simulink model "ALL_JP360_DBW_V6_5_1103"  (R2022a)
settings: Solver=FixedStepAuto  StartTime=0.0  StopTime=inf  FixedStep=0.01  RelTol=1e-3  EnableMultiTasking=on
model workspace (MAT data in the model file):
  g = 9.8
undefined symbols (not defined in the file or in its folder): canChannel, delta_v_p, IPM_Line_C0, IPM_Line_C1, IPM_Line_C2, IPM_Line_C3, M, M_p, MRR_ObjDistX, MRR_ObjDistY, MRR_ObjFusionCamID, MRR_ObjFusionSig, MRR_ObjID, MRR_ObjRelVelX, MRR_ObjRelVelY, MRR_ObjType, MRR_ObjUpdFlg, none, obj_vaild, untracktime, V, videoinput
libraries: canfdmsglib x230, canfdlib x76, slpidlib x24, simulink x18, dspstat3 x14, ctrlSharedLib x1, simulink_extras x1, imaqlib x1, realtime_pacer_lib x1, dspvision x1, visionsinks x1
(part 44 of 55)

== system ALL_JP360_DBW_V6_5_1103/MsgFromCAN/VR_ADCU_MsgFromCAN/VR_ADCU_IPM_Obj_13_0x65C ==
  VR_ADCU_IPM_Obj_13_0x65CFromInData : Inport  OutDataTypeStr=Bus:CAN_FD_MESSAGE_BUS
  Bus Creator : BusCreator  Inputs=18  OutDataTypeStr=Bus:VR_ADCU_IPM_Obj_13_0x65C  NonVirtualBus=on
  CAN FD Unpack : canfdmsglib/CAN FD Unpack  CANdbFile=HiFire_T360_P789_1R1V_Pri_Matrix_CAN_V2.3_20220810.dbc  MsgList=(none)  MsgName=IPM_Obj_13_0x65C  ProtocolMode=CAN FD  MsgIDType=Standard (11-bit identifier)  MsgIdentifier=1628  MsgLength=32  SignalInfo={'IPM_ObjBlockCounter_13','13','11','BE','unsigned','Standard','0','1','0','0','2047';'IPM_ObjDistX_13','58','12','BE','unsigned','Standard','0','0.0625','0','0','254.9375';'IPM_ObjDistY_13','76','14','BE','unsigned','Standard','0','0.0078125','-64','-64','63.9922';'IPM_ObjID_13','16','8','BE','unsigned','Standard','0','1','0','0','255';'IPM_ObjRelAccelX_13','104','10','BE','unsigned','Standard','0','0.03125','-16','-16','15.9688';'IPM_ObjRelAccelY_13','126','10','BE','unsigned','Standard','0','0.03125','-16','-16','15.9688';'IPM_ObjRelVelX_13','95','13','BE','unsigned','Standard','0','0.03125','-128','-128','127.9688';'IPM_ObjRelVelY_13','98','13','BE','unsigned','Standard','0','0.03125','-128','-128','127.9688';'IPM_ObjType_13','54','4','BE','unsigned','Standard','0','1','0','0','15';'IPM_Obj_13_Checksum','248','16','BE','unsigned','Standard','0','1','0','0','65535';'IPM_Obj_13_MsgCounter','232','4','BE','unsigned','Standard','0','1','0','0','15';'IPM_Object_Age_13','37','11','BE','unsigned','Standard','0','1','0','0','2047';'IPM_Object_Existence_Probability_13','42','6','BE','unsigned','Standard','0','2','0','0','100';'IPM_Object_Heading_13','132','10','BE','unsigned','Standard','0','0.01','-3.14','-3.14','3.14';'IPM_Object_Height_13','167','9','BE','unsigned','Standard','0','0.01','0','0','5.11';'IPM_Object_Length_13','139','9','BE','unsigned','Standard','0','0.05','0','0','25.5';'IPM_Object_Motion_Status_13','161','3','BE','unsigned','Standard','0','1','0','0','7';'IPM_Object_Width_13','144','11','BE','unsigned','Standard','0','0.01','0','0','12'}  IDPort=off  TimestampPort=off  ErrorPort=off  RemotePort=off  LengthPort=off  StatusPort=off  BRSPort=off  ESIPort=off  DLCPort=off  ApplyMinMax=off
      settings: SourceProductBaseCode=ME,XP,VN  DataFormat=CANdb specified signals
  Data Type Conversion1 : DataTypeConversion  OutDataTypeStr=int16  SaturateOnIntegerOverflow=off  RndMeth=Floor
  Data Type Conversion10 : DataTypeConversion  OutDataTypeStr=uint16  SaturateOnIntegerOverflow=off  RndMeth=Floor
  Data Type Conversion{9,11,13,17} (4 alike) : DataTypeConversion  OutDataTypeStr=int8  SaturateOnIntegerOverflow=off  RndMeth=Floor
  Data Type Conversion12 : DataTypeConversion  OutDataTypeStr=int16  SaturateOnIntegerOverflow=off  RndMeth=Floor
  Data Type Conversion{2..3,5..8,14..16,18} (10 alike) : DataTypeConversion  OutDataTypeStr=single  SaturateOnIntegerOverflow=off  RndMeth=Floor
  Data Type Conversion4 : DataTypeConversion  OutDataTypeStr=uint8  SaturateOnIntegerOverflow=off  RndMeth=Floor
  VR_ADCU_IPM_Obj_13_0x65CFromOutData : Outport  OutDataTypeStr=Bus:VR_ADCU_IPM_Obj_13_0x65C
  wires:
  CAN FD Unpack/1 -> Data Type Conversion1/1
  CAN FD Unpack/2 -> Data Type Conversion2/1
  CAN FD Unpack/3 -> Data Type Conversion3/1
  CAN FD Unpack/4 -> Data Type Conversion4/1
  CAN FD Unpack/5 -> Data Type Conversion5/1
  CAN FD Unpack/6 -> Data Type Conversion6/1
  CAN FD Unpack/7 -> Data Type Conversion7/1
  CAN FD Unpack/8 -> Data Type Conversion8/1
  CAN FD Unpack/9 -> Data Type Conversion9/1
  CAN FD Unpack/10 -> Data Type Conversion10/1
  CAN FD Unpack/11 -> Data Type Conversion11/1
  CAN FD Unpack/12 -> Data Type Conversion12/1
  CAN FD Unpack/13 -> Data Type Conversion13/1
  CAN FD Unpack/14 -> Data Type Conversion14/1
  CAN FD Unpack/15 -> Data Type Conversion15/1
  CAN FD Unpack/16 -> Data Type Conversion16/1
  CAN FD Unpack/17 -> Data Type Conversion17/1
  CAN FD Unpack/18 -> Data Type Conversion18/1
  Data Type Conversion1/1 -> Bus Creator/1  "IPM_ObjBlockCounter_13"
  Data Type Conversion2/1 -> Bus Creator/2  "IPM_ObjDistX_13"
  Data Type Conversion3/1 -> Bus Creator/3  "IPM_ObjDistY_13"
  Data Type Conversion4/1 -> Bus Creator/4  "IPM_ObjID_13"
  Data Type Conversion5/1 -> Bus Creator/5  "IPM_ObjRelAccelX_13"
  Data Type Conversion6/1 -> Bus Creator/6  "IPM_ObjRelAccelY_13"
  Data Type Conversion7/1 -> Bus Creator/7  "IPM_ObjRelVelX_13"
  Data Type Conversion8/1 -> Bus Creator/8  "IPM_ObjRelVelY_13"
  Data Type Conversion9/1 -> Bus Creator/9  "IPM_ObjType_13"
  Data Type Conversion10/1 -> Bus Creator/10  "IPM_Obj_13_Checksum"
  Data Type Conversion11/1 -> Bus Creator/11  "IPM_Obj_13_MsgCounter"
  Data Type Conversion12/1 -> Bus Creator/12  "IPM_Object_Age_13"
  Data Type Conversion13/1 -> Bus Creator/13  "IPM_Object_Existence_Probability_13"
  Data Type Conversion14/1 -> Bus Creator/14  "IPM_Object_Heading_13"
  Data Type Conversion15/1 -> Bus Creator/15  "IPM_Object_Height_13"
  Data Type Conversion16/1 -> Bus Creator/16  "IPM_Object_Length_13"
  Data Type Conversion17/1 -> Bus Creator/17  "IPM_Object_Motion_Status_13"
  Data Type Conversion18/1 -> Bus Creator/18  "IPM_Object_Width_13"
  Bus Creator/1 -> VR_ADCU_IPM_Obj_13_0x65CFromOutData/1  "VR_ADCU_IPM_Obj_13_0x65CFromOutData"
  VR_ADCU_IPM_Obj_13_0x65CFromInData/1 -> CAN FD Unpack/1  "VR_ADCU_IPM_Obj_13_0x65CFromInData"

== system ALL_JP360_DBW_V6_5_1103/MsgFromCAN/VR_ADCU_MsgFromCAN/VR_ADCU_IPM_Obj_14_0x65D ==
  VR_ADCU_IPM_Obj_14_0x65DFromInData : Inport  OutDataTypeStr=Bus:CAN_FD_MESSAGE_BUS
  Bus Creator : BusCreator  Inputs=18  OutDataTypeStr=Bus:VR_ADCU_IPM_Obj_14_0x65D  NonVirtualBus=on
  CAN FD Unpack : canfdmsglib/CAN FD Unpack  CANdbFile=HiFire_T360_P789_1R1V_Pri_Matrix_CAN_V2.3_20220810.dbc  MsgList=(none)  MsgName=IPM_Obj_14_0x65D  ProtocolMode=CAN FD  MsgIDType=Standard (11-bit identifier)  MsgIdentifier=1629  MsgLength=32  SignalInfo={'IPM_ObjBlockCounter_14','13','11','BE','unsigned','Standard','0','1','0','0','2047';'IPM_ObjDistX_14','58','12','BE','unsigned','Standard','0','0.0625','0','0','254.9375';'IPM_ObjDistY_14','76','14','BE','unsigned','Standard','0','0.0078125','-64','-64','63.9922';'IPM_ObjID_14','16','8','BE','unsigned','Standard','0','1','0','0','255';'IPM_ObjRelAccelX_14','104','10','BE','unsigned','Standard','0','0.03125','-16','-16','15.9688';'IPM_ObjRelAccelY_14','126','10','BE','unsigned','Standard','0','0.03125','-16','-16','15.9688';'IPM_ObjRelVelX_14','95','13','BE','unsigned','Standard','0','0.03125','-128','-128','127.9688';'IPM_ObjRelVelY_14','98','13','BE','unsigned','Standard','0','0.03125','-128','-128','127.9688';'IPM_ObjType_14','54','4','BE','unsigned','Standard','0','1','0','0','15';'IPM_Obj_14_Checksum','248','16','BE','unsigned','Standard','0','1','0','0','65535';'IPM_Obj_14_MsgCounter','232','4','BE','unsigned','Standard','0','1','0','0','15';'IPM_Object_Age_14','37','11','BE','unsigned','Standard','0','1','0','0','2047';'IPM_Object_Existence_Probability_14','42','6','BE','unsigned','Standard','0','2','0','0','100';'IPM_Object_Heading_14','132','10','BE','unsigned','Standard','0','0.01','-3.14','-3.14','3.14';'IPM_Object_Height_14','167','9','BE','unsigned','Standard','0','0.01','0','0','5.11';'IPM_Object_Length_14','139','9','BE','unsigned','Standard','0','0.05','0','0','25.5';'IPM_Object_Motion_Status_14','161','3','BE','unsigned','Standard','0','1','0','0','7';'IPM_Object_Width_14','144','11','BE','unsigned','Standard','0','0.01','0','0','12'}  IDPort=off  TimestampPort=off  ErrorPort=off  RemotePort=off  LengthPort=off  StatusPort=off  BRSPort=off  ESIPort=off  DLCPort=off  ApplyMinMax=off
      settings: SourceProductBaseCode=ME,XP,VN  DataFormat=CANdb specified signals
  Data Type Conversion1 : DataTypeConversion  OutDataTypeStr=int16  SaturateOnIntegerOverflow=off  RndMeth=Floor
  Data Type Conversion10 : DataTypeConversion  OutDataTypeStr=uint16  SaturateOnIntegerOverflow=off  RndMeth=Floor
  Data Type Conversion{9,11,13,17} (4 alike) : DataTypeConversion  OutDataTypeStr=int8  SaturateOnIntegerOverflow=off  RndMeth=Floor
  Data Type Conversion12 : DataTypeConversion  OutDataTypeStr=int16  SaturateOnIntegerOverflow=off  RndMeth=Floor
  Data Type Conversion{2..3,5..8,14..16,18} (10 alike) : DataTypeConversion  OutDataTypeStr=single  SaturateOnIntegerOverflow=off  RndMeth=Floor
  Data Type Conversion4 : DataTypeConversion  OutDataTypeStr=uint8  SaturateOnIntegerOverflow=off  RndMeth=Floor
  VR_ADCU_IPM_Obj_14_0x65DFromOutData : Outport  OutDataTypeStr=Bus:VR_ADCU_IPM_Obj_14_0x65D
  wires:
  CAN FD Unpack/1 -> Data Type Conversion1/1
  CAN FD Unpack/2 -> Data Type Conversion2/1
  CAN FD Unpack/3 -> Data Type Conversion3/1
  CAN FD Unpack/4 -> Data Type Conversion4/1
  CAN FD Unpack/5 -> Data Type Conversion5/1
  CAN FD Unpack/6 -> Data Type Conversion6/1
  CAN FD Unpack/7 -> Data Type Conversion7/1
  CAN FD Unpack/8 -> Data Type Conversion8/1
  CAN FD Unpack/9 -> Data Type Conversion9/1
  CAN FD Unpack/10 -> Data Type Conversion10/1
  CAN FD Unpack/11 -> Data Type Conversion11/1
  CAN FD Unpack/12 -> Data Type Conversion12/1
  CAN FD Unpack/13 -> Data Type Conversion13/1
  CAN FD Unpack/14 -> Data Type Conversion14/1
  CAN FD Unpack/15 -> Data Type Conversion15/1
  CAN FD Unpack/16 -> Data Type Conversion16/1
  CAN FD Unpack/17 -> Data Type Conversion17/1
  CAN FD Unpack/18 -> Data Type Conversion18/1
  Data Type Conversion1/1 -> Bus Creator/1  "IPM_ObjBlockCounter_14"
  Data Type Conversion2/1 -> Bus Creator/2  "IPM_ObjDistX_14"
  Data Type Conversion3/1 -> Bus Creator/3  "IPM_ObjDistY_14"
  Data Type Conversion4/1 -> Bus Creator/4  "IPM_ObjID_14"
  Data Type Conversion5/1 -> Bus Creator/5  "IPM_ObjRelAccelX_14"
  Data Type Conversion6/1 -> Bus Creator/6  "IPM_ObjRelAccelY_14"
  Data Type Conversion7/1 -> Bus Creator/7  "IPM_ObjRelVelX_14"
  Data Type Conversion8/1 -> Bus Creator/8  "IPM_ObjRelVelY_14"
  Data Type Conversion9/1 -> Bus Creator/9  "IPM_ObjType_14"
  Data Type Conversion10/1 -> Bus Creator/10  "IPM_Obj_14_Checksum"
  Data Type Conversion11/1 -> Bus Creator/11  "IPM_Obj_14_MsgCounter"
  Data Type Conversion12/1 -> Bus Creator/12  "IPM_Object_Age_14"
  Data Type Conversion13/1 -> Bus Creator/13  "IPM_Object_Existence_Probability_14"
  Data Type Conversion14/1 -> Bus Creator/14  "IPM_Object_Heading_14"
  Data Type Conversion15/1 -> Bus Creator/15  "IPM_Object_Height_14"
  Data Type Conversion16/1 -> Bus Creator/16  "IPM_Object_Length_14"
  Data Type Conversion17/1 -> Bus Creator/17  "IPM_Object_Motion_Status_14"
  Data Type Conversion18/1 -> Bus Creator/18  "IPM_Object_Width_14"
  Bus Creator/1 -> VR_ADCU_IPM_Obj_14_0x65DFromOutData/1  "VR_ADCU_IPM_Obj_14_0x65DFromOutData"
  VR_ADCU_IPM_Obj_14_0x65DFromInData/1 -> CAN FD Unpack/1  "VR_ADCU_IPM_Obj_14_0x65DFromInData"

== system ALL_JP360_DBW_V6_5_1103/MsgFromCAN/VR_ADCU_MsgFromCAN/VR_ADCU_IPM_Obj_15_0x65E ==
  VR_ADCU_IPM_Obj_15_0x65EFromInData : Inport  OutDataTypeStr=Bus:CAN_FD_MESSAGE_BUS
  Bus Creator : BusCreator  Inputs=18  OutDataTypeStr=Bus:VR_ADCU_IPM_Obj_15_0x65E  NonVirtualBus=on
  CAN FD Unpack : canfdmsglib/CAN FD Unpack  CANdbFile=HiFire_T360_P789_1R1V_Pri_Matrix_CAN_V2.3_20220810.dbc  MsgList=(none)  MsgName=IPM_Obj_15_0x65E  ProtocolMode=CAN FD  MsgIDType=Standard (11-bit identifier)  MsgIdentifier=1630  MsgLength=32  SignalInfo={'IPM_ObjBlockCounter_15','13','11','BE','unsigned','Standard','0','1','0','0','2047';'IPM_ObjDistX_15','58','12','BE','unsigned','Standard','0','0.0625','0','0','254.9375';'IPM_ObjDistY_15','76','14','BE','unsigned','Standard','0','0.0078125','-64','-64','63.9922';'IPM_ObjID_15','16','8','BE','unsigned','Standard','0','1','0','0','255';'IPM_ObjRelAccelX_15','104','10','BE','unsigned','Standard','0','0.03125','-16','-16','15.9688';'IPM_ObjRelAccelY_15','126','10','BE','unsigned','Standard','0','0.03125','-16','-16','15.9688';'IPM_ObjRelVelX_15','95','13','BE','unsigned','Standard','0','0.03125','-128','-128','127.9688';'IPM_ObjRelVelY_15','98','13','BE','unsigned','Standard','0','0.03125','-128','-128','127.9688';'IPM_ObjType_15','54','4','BE','unsigned','Standard','0','1','0','0','15';'IPM_Obj_15_Checksum','248','16','BE','unsigned','Standard','0','1','0','0','65535';'IPM_Obj_15_MsgCounter','232','4','BE','unsigned','Standard','0','1','0','0','15';'IPM_Object_Age_15','37','11','BE','unsigned','Standard','0','1','0','0','2047';'IPM_Object_Existence_Probability_15','42','6','BE','unsigned','Standard','0','2','0','0','100';'IPM_Object_Heading_15','132','10','BE','unsigned','Standard','0','0.01','-3.14','-3.14','3.14';'IPM_Object_Height_15','167','9','BE','unsigned','Standard','0','0.01','0','0','5.11';'IPM_Object_Length_15','139','9','BE','unsigned','Standard','0','0.05','0','0','25.5';'IPM_Object_Motion_Status_15','161','3','BE','unsigned','Standard','0','1','0','0','7';'IPM_Object_Width_15','144','11','BE','unsigned','Standard','0','0.01','0','0','12'}  IDPort=off  TimestampPort=off  ErrorPort=off  RemotePort=off  LengthPort=off  StatusPort=off  BRSPort=off  ESIPort=off  DLCPort=off  ApplyMinMax=off
      settings: SourceProductBaseCode=ME,XP,VN  DataFormat=CANdb specified signals
  Data Type Conversion1 : DataTypeConversion  OutDataTypeStr=int16  SaturateOnIntegerOverflow=off  RndMeth=Floor
  Data Type Conversion10 : DataTypeConversion  OutDataTypeStr=uint16  SaturateOnIntegerOverflow=off  RndMeth=Floor
  Data Type Conversion{9,11,13,17} (4 alike) : DataTypeConversion  OutDataTypeStr=int8  SaturateOnIntegerOverflow=off  RndMeth=Floor
  Data Type Conversion12 : DataTypeConversion  OutDataTypeStr=int16  SaturateOnIntegerOverflow=off  RndMeth=Floor
  Data Type Conversion{2..3,5..8,14..16,18} (10 alike) : DataTypeConversion  OutDataTypeStr=single  SaturateOnIntegerOverflow=off  RndMeth=Floor
  Data Type Conversion4 : DataTypeConversion  OutDataTypeStr=uint8  SaturateOnIntegerOverflow=off  RndMeth=Floor
  VR_ADCU_IPM_Obj_15_0x65EFromOutData : Outport  OutDataTypeStr=Bus:VR_ADCU_IPM_Obj_15_0x65E
  wires:
  CAN FD Unpack/1 -> Data Type Conversion1/1
  CAN FD Unpack/2 -> Data Type Conversion2/1
  CAN FD Unpack/3 -> Data Type Conversion3/1
  CAN FD Unpack/4 -> Data Type Conversion4/1
  CAN FD Unpack/5 -> Data Type Conversion5/1
  CAN FD Unpack/6 -> Data Type Conversion6/1
  CAN FD Unpack/7 -> Data Type Conversion7/1
  CAN FD Unpack/8 -> Data Type Conversion8/1
  CAN FD Unpack/9 -> Data Type Conversion9/1
  CAN FD Unpack/10 -> Data Type Conversion10/1
  CAN FD Unpack/11 -> Data Type Conversion11/1
  CAN FD Unpack/12 -> Data Type Conversion12/1
  CAN FD Unpack/13 -> Data Type Conversion13/1
  CAN FD Unpack/14 -> Data Type Conversion14/1
  CAN FD Unpack/15 -> Data Type Conversion15/1
  CAN FD Unpack/16 -> Data Type Conversion16/1
  CAN FD Unpack/17 -> Data Type Conversion17/1
  CAN FD Unpack/18 -> Data Type Conversion18/1
  Data Type Conversion1/1 -> Bus Creator/1  "IPM_ObjBlockCounter_15"
  Data Type Conversion2/1 -> Bus Creator/2  "IPM_ObjDistX_15"
  Data Type Conversion3/1 -> Bus Creator/3  "IPM_ObjDistY_15"
  Data Type Conversion4/1 -> Bus Creator/4  "IPM_ObjID_15"
  Data Type Conversion5/1 -> Bus Creator/5  "IPM_ObjRelAccelX_15"
  Data Type Conversion6/1 -> Bus Creator/6  "IPM_ObjRelAccelY_15"
  Data Type Conversion7/1 -> Bus Creator/7  "IPM_ObjRelVelX_15"
  Data Type Conversion8/1 -> Bus Creator/8  "IPM_ObjRelVelY_15"
  Data Type Conversion9/1 -> Bus Creator/9  "IPM_ObjType_15"
  Data Type Conversion10/1 -> Bus Creator/10  "IPM_Obj_15_Checksum"
  Data Type Conversion11/1 -> Bus Creator/11  "IPM_Obj_15_MsgCounter"
  Data Type Conversion12/1 -> Bus Creator/12  "IPM_Object_Age_15"
  Data Type Conversion13/1 -> Bus Creator/13  "IPM_Object_Existence_Probability_15"
  Data Type Conversion14/1 -> Bus Creator/14  "IPM_Object_Heading_15"
  Data Type Conversion15/1 -> Bus Creator/15  "IPM_Object_Height_15"
  Data Type Conversion16/1 -> Bus Creator/16  "IPM_Object_Length_15"
  Data Type Conversion17/1 -> Bus Creator/17  "IPM_Object_Motion_Status_15"
  Data Type Conversion18/1 -> Bus Creator/18  "IPM_Object_Width_15"
  Bus Creator/1 -> VR_ADCU_IPM_Obj_15_0x65EFromOutData/1  "VR_ADCU_IPM_Obj_15_0x65EFromOutData"
  VR_ADCU_IPM_Obj_15_0x65EFromInData/1 -> CAN FD Unpack/1  "VR_ADCU_IPM_Obj_15_0x65EFromInData"

== system ALL_JP360_DBW_V6_5_1103/MsgFromCAN/VR_ADCU_MsgFromCAN/VR_ADCU_IPM_Obj_16_0x65F ==
  VR_ADCU_IPM_Obj_16_0x65FFromInData : Inport  OutDataTypeStr=Bus:CAN_FD_MESSAGE_BUS
  Bus Creator : BusCreator  Inputs=18  OutDataTypeStr=Bus:VR_ADCU_IPM_Obj_16_0x65F  NonVirtualBus=on
  CAN FD Unpack : canfdmsglib/CAN FD Unpack  CANdbFile=HiFire_T360_P789_1R1V_Pri_Matrix_CAN_V2.3_20220810.dbc  MsgList=(none)  MsgName=IPM_Obj_16_0x65F  ProtocolMode=CAN FD  MsgIDType=Standard (11-bit identifier)  MsgIdentifier=1631  MsgLength=32  SignalInfo={'IPM_ObjBlockCounter_16','13','11','BE','unsigned','Standard','0','1','0','0','2047';'IPM_ObjDistX_16','58','12','BE','unsigned','Standard','0','0.0625','0','0','254.9375';'IPM_ObjDistY_16','76','14','BE','unsigned','Standard','0','0.0078125','-64','-64','63.9922';'IPM_ObjID_16','16','8','BE','unsigned','Standard','0','1','0','0','255';'IPM_ObjRelAccelX_16','104','10','BE','unsigned','Standard','0','0.03125','-16','-16','15.9688';'IPM_ObjRelAccelY_16','126','10','BE','unsigned','Standard','0','0.03125','-16','-16','15.9688';'IPM_ObjRelVelX_16','95','13','BE','unsigned','Standard','0','0.03125','-128','-128','127.9688';'IPM_ObjRelVelY_16','98','13','BE','unsigned','Standard','0','0.03125','-128','-128','127.9688';'IPM_ObjType_16','54','4','BE','unsigned','Standard','0','1','0','0','15';'IPM_Obj_16_Checksum','248','16','BE','unsigned','Standard','0','1','0','0','65535';'IPM_Obj_16_MsgCounter','232','4','BE','unsigned','Standard','0','1','0','0','15';'IPM_Object_Age_16','37','11','BE','unsigned','Standard','0','1','0','0','2047';'IPM_Object_Existence_Probability_16','42','6','BE','unsigned','Standard','0','2','0','0','100';'IPM_Object_Heading_16','132','10','BE','unsigned','Standard','0','0.01','-3.14','-3.14','3.14';'IPM_Object_Height_16','167','9','BE','unsigned','Standard','0','0.01','0','0','5.11';'IPM_Object_Length_16','139','9','BE','unsigned','Standard','0','0.05','0','0','25.5';'IPM_Object_Motion_Status_16','161','3','BE','unsigned','Standard','0','1','0','0','7';'IPM_Object_Width_16','144','11','BE','unsigned','Standard','0','0.01','0','0','12'}  IDPort=off  TimestampPort=off  ErrorPort=off  RemotePort=off  LengthPort=off  StatusPort=off  BRSPort=off  ESIPort=off  DLCPort=off  ApplyMinMax=off
      settings: SourceProductBaseCode=ME,XP,VN  DataFormat=CANdb specified signals
  Data Type Conversion1 : DataTypeConversion  OutDataTypeStr=int16  SaturateOnIntegerOverflow=off  RndMeth=Floor
  Data Type Conversion10 : DataTypeConversion  OutDataTypeStr=uint16  SaturateOnIntegerOverflow=off  RndMeth=Floor
  Data Type Conversion{9,11,13,17} (4 alike) : DataTypeConversion  OutDataTypeStr=int8  SaturateOnIntegerOverflow=off  RndMeth=Floor
  Data Type Conversion12 : DataTypeConversion  OutDataTypeStr=int16  SaturateOnIntegerOverflow=off  RndMeth=Floor
  Data Type Conversion{2..3,5..8,14..16,18} (10 alike) : DataTypeConversion  OutDataTypeStr=single  SaturateOnIntegerOverflow=off  RndMeth=Floor
  Data Type Conversion4 : DataTypeConversion  OutDataTypeStr=uint8  SaturateOnIntegerOverflow=off  RndMeth=Floor
  VR_ADCU_IPM_Obj_16_0x65FFromOutData : Outport  OutDataTypeStr=Bus:VR_ADCU_IPM_Obj_16_0x65F
  wires:
  CAN FD Unpack/1 -> Data Type Conversion1/1
  CAN FD Unpack/2 -> Data Type Conversion2/1
  CAN FD Unpack/3 -> Data Type Conversion3/1
  CAN FD Unpack/4 -> Data Type Conversion4/1
  CAN FD Unpack/5 -> Data Type Conversion5/1
  CAN FD Unpack/6 -> Data Type Conversion6/1
  CAN FD Unpack/7 -> Data Type Conversion7/1
  CAN FD Unpack/8 -> Data Type Conversion8/1
  CAN FD Unpack/9 -> Data Type Conversion9/1
  CAN FD Unpack/10 -> Data Type Conversion10/1
  CAN FD Unpack/11 -> Data Type Conversion11/1
  CAN FD Unpack/12 -> Data Type Conversion12/1
  CAN FD Unpack/13 -> Data Type Conversion13/1
  CAN FD Unpack/14 -> Data Type Conversion14/1
  CAN FD Unpack/15 -> Data Type Conversion15/1
  CAN FD Unpack/16 -> Data Type Conversion16/1
  CAN FD Unpack/17 -> Data Type Conversion17/1
  CAN FD Unpack/18 -> Data Type Conversion18/1
  Data Type Conversion1/1 -> Bus Creator/1  "IPM_ObjBlockCounter_16"
  Data Type Conversion2/1 -> Bus Creator/2  "IPM_ObjDistX_16"
  Data Type Conversion3/1 -> Bus Creator/3  "IPM_ObjDistY_16"
  Data Type Conversion4/1 -> Bus Creator/4  "IPM_ObjID_16"
  Data Type Conversion5/1 -> Bus Creator/5  "IPM_ObjRelAccelX_16"
  Data Type Conversion6/1 -> Bus Creator/6  "IPM_ObjRelAccelY_16"
  Data Type Conversion7/1 -> Bus Creator/7  "IPM_ObjRelVelX_16"
  Data Type Conversion8/1 -> Bus Creator/8  "IPM_ObjRelVelY_16"
  Data Type Conversion9/1 -> Bus Creator/9  "IPM_ObjType_16"
  Data Type Conversion10/1 -> Bus Creator/10  "IPM_Obj_16_Checksum"
  Data Type Conversion11/1 -> Bus Creator/11  "IPM_Obj_16_MsgCounter"
  Data Type Conversion12/1 -> Bus Creator/12  "IPM_Object_Age_16"
  Data Type Conversion13/1 -> Bus Creator/13  "IPM_Object_Existence_Probability_16"
  Data Type Conversion14/1 -> Bus Creator/14  "IPM_Object_Heading_16"
  Data Type Conversion15/1 -> Bus Creator/15  "IPM_Object_Height_16"
  Data Type Conversion16/1 -> Bus Creator/16  "IPM_Object_Length_16"
  Data Type Conversion17/1 -> Bus Creator/17  "IPM_Object_Motion_Status_16"
  Data Type Conversion18/1 -> Bus Creator/18  "IPM_Object_Width_16"
  Bus Creator/1 -> VR_ADCU_IPM_Obj_16_0x65FFromOutData/1  "VR_ADCU_IPM_Obj_16_0x65FFromOutData"
  VR_ADCU_IPM_Obj_16_0x65FFromInData/1 -> CAN FD Unpack/1  "VR_ADCU_IPM_Obj_16_0x65FFromInData"

== system ALL_JP360_DBW_V6_5_1103/MsgFromCAN/VR_ADCU_MsgFromCAN/VR_ADCU_IPM_Obj_17_0x660 ==
  VR_ADCU_IPM_Obj_17_0x660FromInData : Inport  OutDataTypeStr=Bus:CAN_FD_MESSAGE_BUS
  Bus Creator : BusCreator  Inputs=18  OutDataTypeStr=Bus:VR_ADCU_IPM_Obj_17_0x660  NonVirtualBus=on
  CAN FD Unpack : canfdmsglib/CAN FD Unpack  CANdbFile=HiFire_T360_P789_1R1V_Pri_Matrix_CAN_V2.3_20220810.dbc  MsgList=(none)  MsgName=IPM_Obj_17_0x660  ProtocolMode=CAN FD  MsgIDType=Standard (11-bit identifier)  MsgIdentifier=1632  MsgLength=32  SignalInfo={'IPM_ObjBlockCounter_17','13','11','BE','unsigned','Standard','0','1','0','0','2047';'IPM_ObjDistX_17','58','12','BE','unsigned','Standard','0','0.0625','0','0','254.9375';'IPM_ObjDistY_17','76','14','BE','unsigned','Standard','0','0.0078125','-64','-64','63.9922';'IPM_ObjID_17','16','8','BE','unsigned','Standard','0','1','0','0','255';'IPM_ObjRelAccelX_17','104','10','BE','unsigned','Standard','0','0.03125','-16','-16','15.9688';'IPM_ObjRelAccelY_17','126','10','BE','unsigned','Standard','0','0.03125','-16','-16','15.9688';'IPM_ObjRelVelX_17','95','13','BE','unsigned','Standard','0','0.03125','-128','-128','127.9688';'IPM_ObjRelVelY_17','98','13','BE','unsigned','Standard','0','0.03125','-128','-128','127.9688';'IPM_ObjType_17','54','4','BE','unsigned','Standard','0','1','0','0','15';'IPM_Obj_17_Checksum','248','16','BE','unsigned','Standard','0','1','0','0','65535';'IPM_Obj_17_MsgCounter','232','4','BE','unsigned','Standard','0','1','0','0','15';'IPM_Object_Age_17','37','11','BE','unsigned','Standard','0','1','0','0','2047';'IPM_Object_Existence_Probability_17','42','6','BE','unsigned','Standard','0','2','0','0','100';'IPM_Object_Heading_17','132','10','BE','unsigned','Standard','0','0.01','-3.14','-3.14','3.14';'IPM_Object_Height_17','167','9','BE','unsigned','Standard','0','0.01','0','0','5.11';'IPM_Object_Length_17','139','9','BE','unsigned','Standard','0','0.05','0','0','25.5';'IPM_Object_Motion_Status_17','161','3','BE','unsigned','Standard','0','1','0','0','7';'IPM_Object_Width_17','144','11','BE','unsigned','Standard','0','0.01','0','0','12'}  IDPort=off  TimestampPort=off  ErrorPort=off  RemotePort=off  LengthPort=off  StatusPort=off  BRSPort=off  ESIPort=off  DLCPort=off  ApplyMinMax=off
      settings: SourceProductBaseCode=ME,XP,VN  DataFormat=CANdb specified signals
  Data Type Conversion1 : DataTypeConversion  OutDataTypeStr=int16  SaturateOnIntegerOverflow=off  RndMeth=Floor
  Data Type Conversion10 : DataTypeConversion  OutDataTypeStr=uint16  SaturateOnIntegerOverflow=off  RndMeth=Floor
  Data Type Conversion{9,11,13,17} (4 alike) : DataTypeConversion  OutDataTypeStr=int8  SaturateOnIntegerOverflow=off  RndMeth=Floor
  Data Type Conversion12 : DataTypeConversion  OutDataTypeStr=int16  SaturateOnIntegerOverflow=off  RndMeth=Floor
  Data Type Conversion{2..3,5..8,14..16,18} (10 alike) : DataTypeConversion  OutDataTypeStr=single  SaturateOnIntegerOverflow=off  RndMeth=Floor
  Data Type Conversion4 : DataTypeConversion  OutDataTypeStr=uint8  SaturateOnIntegerOverflow=off  RndMeth=Floor
  VR_ADCU_IPM_Obj_17_0x660FromOutData : Outport  OutDataTypeStr=Bus:VR_ADCU_IPM_Obj_17_0x660
  wires:
  CAN FD Unpack/1 -> Data Type Conversion1/1
  CAN FD Unpack/2 -> Data Type Conversion2/1
  CAN FD Unpack/3 -> Data Type Conversion3/1
  CAN FD Unpack/4 -> Data Type Conversion4/1
  CAN FD Unpack/5 -> Data Type Conversion5/1
  CAN FD Unpack/6 -> Data Type Conversion6/1
  CAN FD Unpack/7 -> Data Type Conversion7/1
  CAN FD Unpack/8 -> Data Type Conversion8/1
  CAN FD Unpack/9 -> Data Type Conversion9/1
  CAN FD Unpack/10 -> Data Type Conversion10/1
  CAN FD Unpack/11 -> Data Type Conversion11/1
  CAN FD Unpack/12 -> Data Type Conversion12/1
  CAN FD Unpack/13 -> Data Type Conversion13/1
  CAN FD Unpack/14 -> Data Type Conversion14/1
  CAN FD Unpack/15 -> Data Type Conversion15/1
  CAN FD Unpack/16 -> Data Type Conversion16/1
  CAN FD Unpack/17 -> Data Type Conversion17/1
  CAN FD Unpack/18 -> Data Type Conversion18/1
  Data Type Conversion1/1 -> Bus Creator/1  "IPM_ObjBlockCounter_17"
  Data Type Conversion2/1 -> Bus Creator/2  "IPM_ObjDistX_17"
  Data Type Conversion3/1 -> Bus Creator/3  "IPM_ObjDistY_17"
  Data Type Conversion4/1 -> Bus Creator/4  "IPM_ObjID_17"
  Data Type Conversion5/1 -> Bus Creator/5  "IPM_ObjRelAccelX_17"
  Data Type Conversion6/1 -> Bus Creator/6  "IPM_ObjRelAccelY_17"
  Data Type Conversion7/1 -> Bus Creator/7  "IPM_ObjRelVelX_17"
  Data Type Conversion8/1 -> Bus Creator/8  "IPM_ObjRelVelY_17"
  Data Type Conversion9/1 -> Bus Creator/9  "IPM_ObjType_17"
  Data Type Conversion10/1 -> Bus Creator/10  "IPM_Obj_17_Checksum"
  Data Type Conversion11/1 -> Bus Creator/11  "IPM_Obj_17_MsgCounter"
  Data Type Conversion12/1 -> Bus Creator/12  "IPM_Object_Age_17"
  Data Type Conversion13/1 -> Bus Creator/13  "IPM_Object_Existence_Probability_17"
  Data Type Conversion14/1 -> Bus Creator/14  "IPM_Object_Heading_17"
  Data Type Conversion15/1 -> Bus Creator/15  "IPM_Object_Height_17"
  Data Type Conversion16/1 -> Bus Creator/16  "IPM_Object_Length_17"
  Data Type Conversion17/1 -> Bus Creator/17  "IPM_Object_Motion_Status_17"
  Data Type Conversion18/1 -> Bus Creator/18  "IPM_Object_Width_17"
  Bus Creator/1 -> VR_ADCU_IPM_Obj_17_0x660FromOutData/1  "VR_ADCU_IPM_Obj_17_0x660FromOutData"
  VR_ADCU_IPM_Obj_17_0x660FromInData/1 -> CAN FD Unpack/1  "VR_ADCU_IPM_Obj_17_0x660FromInData"

== system ALL_JP360_DBW_V6_5_1103/MsgFromCAN/VR_ADCU_MsgFromCAN/VR_ADCU_IPM_Obj_18_0x661 ==
  VR_ADCU_IPM_Obj_18_0x661FromInData : Inport  OutDataTypeStr=Bus:CAN_FD_MESSAGE_BUS
  Bus Creator : BusCreator  Inputs=18  OutDataTypeStr=Bus:VR_ADCU_IPM_Obj_18_0x661  NonVirtualBus=on
  CAN FD Unpack : canfdmsglib/CAN FD Unpack  CANdbFile=HiFire_T360_P789_1R1V_Pri_Matrix_CAN_V2.3_20220810.dbc  MsgList=(none)  MsgName=IPM_Obj_18_0x661  ProtocolMode=CAN FD  MsgIDType=Standard (11-bit identifier)  MsgIdentifier=1633  MsgLength=32  SignalInfo={'IPM_ObjBlockCounter_18','13','11','BE','unsigned','Standard','0','1','0','0','2047';'IPM_ObjDistX_18','58','12','BE','unsigned','Standard','0','0.0625','0','0','254.9375';'IPM_ObjDistY_18','76','14','BE','unsigned','Standard','0','0.0078125','-64','-64','63.9922';'IPM_ObjID_18','16','8','BE','unsigned','Standard','0','1','0','0','255';'IPM_ObjRelAccelX_18','104','10','BE','unsigned','Standard','0','0.03125','-16','-16','15.9688';'IPM_ObjRelAccelY_18','126','10','BE','unsigned','Standard','0','0.03125','-16','-16','15.9688';'IPM_ObjRelVelX_18','95','13','BE','unsigned','Standard','0','0.03125','-128','-128','127.9688';'IPM_ObjRelVelY_18','98','13','BE','unsigned','Standard','0','0.03125','-128','-128','127.9688';'IPM_ObjType_18','54','4','BE','unsigned','Standard','0','1','0','0','15';'IPM_Obj_18_Checksum','248','16','BE','unsigned','Standard','0','1','0','0','65535';'IPM_Obj_18_MsgCounter','232','4','BE','unsigned','Standard','0','1','0','0','15';'IPM_Object_Age_18','37','11','BE','unsigned','Standard','0','1','0','0','2047';'IPM_Object_Existence_Probability_18','42','6','BE','unsigned','Standard','0','2','0','0','100';'IPM_Object_Heading_18','132','10','BE','unsigned','Standard','0','0.01','-3.14','-3.14','3.14';'IPM_Object_Height_18','167','9','BE','unsigned','Standard','0','0.01','0','0','5.11';'IPM_Object_Length_18','139','9','BE','unsigned','Standard','0','0.05','0','0','25.5';'IPM_Object_Motion_Status_18','161','3','BE','unsigned','Standard','0','1','0','0','7';'IPM_Object_Width_18','144','11','BE','unsigned','Standard','0','0.01','0','0','12'}  IDPort=off  TimestampPort=off  ErrorPort=off  RemotePort=off  LengthPort=off  StatusPort=off  BRSPort=off  ESIPort=off  DLCPort=off  ApplyMinMax=off
      settings: SourceProductBaseCode=ME,XP,VN  DataFormat=CANdb specified signals
  Data Type Conversion1 : DataTypeConversion  OutDataTypeStr=int16  SaturateOnIntegerOverflow=off  RndMeth=Floor
  Data Type Conversion10 : DataTypeConversion  OutDataTypeStr=uint16  SaturateOnIntegerOverflow=off  RndMeth=Floor
  Data Type Conversion{9,11,13,17} (4 alike) : DataTypeConversion  OutDataTypeStr=int8  SaturateOnIntegerOverflow=off  RndMeth=Floor
  Data Type Conversion12 : DataTypeConversion  OutDataTypeStr=int16  SaturateOnIntegerOverflow=off  RndMeth=Floor
  Data Type Conversion{2..3,5..8,14..16,18} (10 alike) : DataTypeConversion  OutDataTypeStr=single  SaturateOnIntegerOverflow=off  RndMeth=Floor
  Data Type Conversion4 : DataTypeConversion  OutDataTypeStr=uint8  SaturateOnIntegerOverflow=off  RndMeth=Floor
  VR_ADCU_IPM_Obj_18_0x661FromOutData : Outport  OutDataTypeStr=Bus:VR_ADCU_IPM_Obj_18_0x661
  wires:
  CAN FD Unpack/1 -> Data Type Conversion1/1
  CAN FD Unpack/2 -> Data Type Conversion2/1
  CAN FD Unpack/3 -> Data Type Conversion3/1
  CAN FD Unpack/4 -> Data Type Conversion4/1
  CAN FD Unpack/5 -> Data Type Conversion5/1
  CAN FD Unpack/6 -> Data Type Conversion6/1
  CAN FD Unpack/7 -> Data Type Conversion7/1
  CAN FD Unpack/8 -> Data Type Conversion8/1
  CAN FD Unpack/9 -> Data Type Conversion9/1
  CAN FD Unpack/10 -> Data Type Conversion10/1
  CAN FD Unpack/11 -> Data Type Conversion11/1
  CAN FD Unpack/12 -> Data Type Conversion12/1
  CAN FD Unpack/13 -> Data Type Conversion13/1
  CAN FD Unpack/14 -> Data Type Conversion14/1
  CAN FD Unpack/15 -> Data Type Conversion15/1
  CAN FD Unpack/16 -> Data Type Conversion16/1
  CAN FD Unpack/17 -> Data Type Conversion17/1
  CAN FD Unpack/18 -> Data Type Conversion18/1
  Data Type Conversion1/1 -> Bus Creator/1  "IPM_ObjBlockCounter_18"
  Data Type Conversion2/1 -> Bus Creator/2  "IPM_ObjDistX_18"
  Data Type Conversion3/1 -> Bus Creator/3  "IPM_ObjDistY_18"
  Data Type Conversion4/1 -> Bus Creator/4  "IPM_ObjID_18"
  Data Type Conversion5/1 -> Bus Creator/5  "IPM_ObjRelAccelX_18"
  Data Type Conversion6/1 -> Bus Creator/6  "IPM_ObjRelAccelY_18"
  Data Type Conversion7/1 -> Bus Creator/7  "IPM_ObjRelVelX_18"
  Data Type Conversion8/1 -> Bus Creator/8  "IPM_ObjRelVelY_18"
  Data Type Conversion9/1 -> Bus Creator/9  "IPM_ObjType_18"
  Data Type Conversion10/1 -> Bus Creator/10  "IPM_Obj_18_Checksum"
  Data Type Conversion11/1 -> Bus Creator/11  "IPM_Obj_18_MsgCounter"
  Data Type Conversion12/1 -> Bus Creator/12  "IPM_Object_Age_18"
  Data Type Conversion13/1 -> Bus Creator/13  "IPM_Object_Existence_Probability_18"
  Data Type Conversion14/1 -> Bus Creator/14  "IPM_Object_Heading_18"
  Data Type Conversion15/1 -> Bus Creator/15  "IPM_Object_Height_18"
  Data Type Conversion16/1 -> Bus Creator/16  "IPM_Object_Length_18"
  Data Type Conversion17/1 -> Bus Creator/17  "IPM_Object_Motion_Status_18"
  Data Type Conversion18/1 -> Bus Creator/18  "IPM_Object_Width_18"
  Bus Creator/1 -> VR_ADCU_IPM_Obj_18_0x661FromOutData/1  "VR_ADCU_IPM_Obj_18_0x661FromOutData"
  VR_ADCU_IPM_Obj_18_0x661FromInData/1 -> CAN FD Unpack/1  "VR_ADCU_IPM_Obj_18_0x661FromInData"

== system ALL_JP360_DBW_V6_5_1103/MsgFromCAN/VR_ADCU_MsgFromCAN/VR_ADCU_IPM_Obj_19_0x662 ==
  VR_ADCU_IPM_Obj_19_0x662FromInData : Inport  OutDataTypeStr=Bus:CAN_FD_MESSAGE_BUS
  Bus Creator : BusCreator  Inputs=18  OutDataTypeStr=Bus:VR_ADCU_IPM_Obj_19_0x662  NonVirtualBus=on
  CAN FD Unpack : canfdmsglib/CAN FD Unpack  CANdbFile=HiFire_T360_P789_1R1V_Pri_Matrix_CAN_V2.3_20220810.dbc  MsgList=(none)  MsgName=IPM_Obj_19_0x662  ProtocolMode=CAN FD  MsgIDType=Standard (11-bit identifier)  MsgIdentifier=1634  MsgLength=32  SignalInfo={'IPM_ObjBlockCounter_19','13','11','BE','unsigned','Standard','0','1','0','0','2047';'IPM_ObjDistX_19','58','12','BE','unsigned','Standard','0','0.0625','0','0','254.9375';'IPM_ObjDistY_19','76','14','BE','unsigned','Standard','0','0.0078125','-64','-64','63.9922';'IPM_ObjID_19','16','8','BE','unsigned','Standard','0','1','0','0','255';'IPM_ObjRelAccelX_19','104','10','BE','unsigned','Standard','0','0.03125','-16','-16','15.9688';'IPM_ObjRelAccelY_19','126','10','BE','unsigned','Standard','0','0.03125','-16','-16','15.9688';'IPM_ObjRelVelX_19','95','13','BE','unsigned','Standard','0','0.03125','-128','-128','127.9688';'IPM_ObjRelVelY_19','98','13','BE','unsigned','Standard','0','0.03125','-128','-128','127.9688';'IPM_ObjType_19','54','4','BE','unsigned','Standard','0','1','0','0','15';'IPM_Obj_19_Checksum','248','16','BE','unsigned','Standard','0','1','0','0','65535';'IPM_Obj_19_MsgCounter','232','4','BE','unsigned','Standard','0','1','0','0','15';'IPM_Object_Age_19','37','11','BE','unsigned','Standard','0','1','0','0','2047';'IPM_Object_Existence_Probability_19','42','6','BE','unsigned','Standard','0','2','0','0','100';'IPM_Object_Heading_19','132','10','BE','unsigned','Standard','0','0.01','-3.14','-3.14','3.14';'IPM_Object_Height_19','167','9','BE','unsigned','Standard','0','0.01','0','0','5.11';'IPM_Object_Length_19','139','9','BE','unsigned','Standard','0','0.05','0','0','25.5';'IPM_Object_Motion_Status_19','161','3','BE','unsigned','Standard','0','1','0','0','7';'IPM_Object_Width_19','144','11','BE','unsigned','Standard','0','0.01','0','0','12'}  IDPort=off  TimestampPort=off  ErrorPort=off  RemotePort=off  LengthPort=off  StatusPort=off  BRSPort=off  ESIPort=off  DLCPort=off  ApplyMinMax=off
      settings: SourceProductBaseCode=ME,XP,VN  DataFormat=CANdb specified signals
  Data Type Conversion1 : DataTypeConversion  OutDataTypeStr=int16  SaturateOnIntegerOverflow=off  RndMeth=Floor
  Data Type Conversion10 : DataTypeConversion  OutDataTypeStr=uint16  SaturateOnIntegerOverflow=off  RndMeth=Floor
  Data Type Conversion{9,11,13,17} (4 alike) : DataTypeConversion  OutDataTypeStr=int8  SaturateOnIntegerOverflow=off  RndMeth=Floor
  Data Type Conversion12 : DataTypeConversion  OutDataTypeStr=int16  SaturateOnIntegerOverflow=off  RndMeth=Floor
  Data Type Conversion{2..3,5..8,14..16,18} (10 alike) : DataTypeConversion  OutDataTypeStr=single  SaturateOnIntegerOverflow=off  RndMeth=Floor
  Data Type Conversion4 : DataTypeConversion  OutDataTypeStr=uint8  SaturateOnIntegerOverflow=off  RndMeth=Floor
  VR_ADCU_IPM_Obj_19_0x662FromOutData : Outport  OutDataTypeStr=Bus:VR_ADCU_IPM_Obj_19_0x662
  wires:
  CAN FD Unpack/1 -> Data Type Conversion1/1
  CAN FD Unpack/2 -> Data Type Conversion2/1
  CAN FD Unpack/3 -> Data Type Conversion3/1
  CAN FD Unpack/4 -> Data Type Conversion4/1
  CAN FD Unpack/5 -> Data Type Conversion5/1
  CAN FD Unpack/6 -> Data Type Conversion6/1
  CAN FD Unpack/7 -> Data Type Conversion7/1
  CAN FD Unpack/8 -> Data Type Conversion8/1
  CAN FD Unpack/9 -> Data Type Conversion9/1
  CAN FD Unpack/10 -> Data Type Conversion10/1
  CAN FD Unpack/11 -> Data Type Conversion11/1
  CAN FD Unpack/12 -> Data Type Conversion12/1
  CAN FD Unpack/13 -> Data Type Conversion13/1
  CAN FD Unpack/14 -> Data Type Conversion14/1
  CAN FD Unpack/15 -> Data Type Conversion15/1
  CAN FD Unpack/16 -> Data Type Conversion16/1
  CAN FD Unpack/17 -> Data Type Conversion17/1
  CAN FD Unpack/18 -> Data Type Conversion18/1
  Data Type Conversion1/1 -> Bus Creator/1  "IPM_ObjBlockCounter_19"
  Data Type Conversion2/1 -> Bus Creator/2  "IPM_ObjDistX_19"
  Data Type Conversion3/1 -> Bus Creator/3  "IPM_ObjDistY_19"
  Data Type Conversion4/1 -> Bus Creator/4  "IPM_ObjID_19"
  Data Type Conversion5/1 -> Bus Creator/5  "IPM_ObjRelAccelX_19"
  Data Type Conversion6/1 -> Bus Creator/6  "IPM_ObjRelAccelY_19"
  Data Type Conversion7/1 -> Bus Creator/7  "IPM_ObjRelVelX_19"
  Data Type Conversion8/1 -> Bus Creator/8  "IPM_ObjRelVelY_19"
  Data Type Conversion9/1 -> Bus Creator/9  "IPM_ObjType_19"
  Data Type Conversion10/1 -> Bus Creator/10  "IPM_Obj_19_Checksum"
  Data Type Conversion11/1 -> Bus Creator/11  "IPM_Obj_19_MsgCounter"
  Data Type Conversion12/1 -> Bus Creator/12  "IPM_Object_Age_19"
  Data Type Conversion13/1 -> Bus Creator/13  "IPM_Object_Existence_Probability_19"
  Data Type Conversion14/1 -> Bus Creator/14  "IPM_Object_Heading_19"
  Data Type Conversion15/1 -> Bus Creator/15  "IPM_Object_Height_19"
  Data Type Conversion16/1 -> Bus Creator/16  "IPM_Object_Length_19"
  Data Type Conversion17/1 -> Bus Creator/17  "IPM_Object_Motion_Status_19"
  Data Type Conversion18/1 -> Bus Creator/18  "IPM_Object_Width_19"
  Bus Creator/1 -> VR_ADCU_IPM_Obj_19_0x662FromOutData/1  "VR_ADCU_IPM_Obj_19_0x662FromOutData"
  VR_ADCU_IPM_Obj_19_0x662FromInData/1 -> CAN FD Unpack/1  "VR_ADCU_IPM_Obj_19_0x662FromInData"

== system ALL_JP360_DBW_V6_5_1103/MsgFromCAN/VR_ADCU_MsgFromCAN/VR_ADCU_IPM_Obj_20_0x663 ==
  VR_ADCU_IPM_Obj_20_0x663FromInData : Inport  OutDataTypeStr=Bus:CAN_FD_MESSAGE_BUS
  Bus Creator : BusCreator  Inputs=18  OutDataTypeStr=Bus:VR_ADCU_IPM_Obj_20_0x663  NonVirtualBus=on
  CAN FD Unpack : canfdmsglib/CAN FD Unpack  CANdbFile=HiFire_T360_P789_1R1V_Pri_Matrix_CAN_V2.3_20220810.dbc  MsgList=(none)  MsgName=IPM_Obj_20_0x663  ProtocolMode=CAN FD  MsgIDType=Standard (11-bit identifier)  MsgIdentifier=1635  MsgLength=32  SignalInfo={'IPM_ObjBlockCounter_20','13','11','BE','unsigned','Standard','0','1','0','0','2047';'IPM_ObjDistX_20','58','12','BE','unsigned','Standard','0','0.0625','0','0','254.9375';'IPM_ObjDistY_20','76','14','BE','unsigned','Standard','0','0.0078125','-64','-64','63.9922';'IPM_ObjID_20','16','8','BE','unsigned','Standard','0','1','0','0','255';'IPM_ObjRelAccelX_20','104','10','BE','unsigned','Standard','0','0.03125','-16','-16','15.9688';'IPM_ObjRelAccelY_20','126','10','BE','unsigned','Standard','0','0.03125','-16','-16','15.9688';'IPM_ObjRelVelX_20','95','13','BE','unsigned','Standard','0','0.03125','-128','-128','127.9688';'IPM_ObjRelVelY_20','98','13','BE','unsigned','Standard','0','0.03125','-128','-128','127.9688';'IPM_ObjType_20','54','4','BE','unsigned','Standard','0','1','0','0','15';'IPM_Obj_20_Checksum','248','16','BE','unsigned','Standard','0','1','0','0','65535';'IPM_Obj_20_MsgCounter','232','4','BE','unsigned','Standard','0','1','0','0','15';'IPM_Object_Age_20','37','11','BE','unsigned','Standard','0','1','0','0','2047';'IPM_Object_Existence_Probability_20','42','6','BE','unsigned','Standard','0','2','0','0','100';'IPM_Object_Heading_20','132','10','BE','unsigned','Standard','0','0.01','-3.14','-3.14','3.14';'IPM_Object_Height_20','167','9','BE','unsigned','Standard','0','0.01','0','0','5.11';'IPM_Object_Length_20','139','9','BE','unsigned','Standard','0','0.05','0','0','25.5';'IPM_Object_Motion_Status_20','161','3','BE','unsigned','Standard','0','1','0','0','7';'IPM_Object_Width_20','144','11','BE','unsigned','Standard','0','0.01','0','0','12'}  IDPort=off  TimestampPort=off  ErrorPort=off  RemotePort=off  LengthPort=off  StatusPort=off  BRSPort=off  ESIPort=off  DLCPort=off  ApplyMinMax=off
      settings: SourceProductBaseCode=ME,XP,VN  DataFormat=CANdb specified signals
  Data Type Conversion1 : DataTypeConversion  OutDataTypeStr=int16  SaturateOnIntegerOverflow=off  RndMeth=Floor
  Data Type Conversion10 : DataTypeConversion  OutDataTypeStr=uint16  SaturateOnIntegerOverflow=off  RndMeth=Floor
  Data Type Conversion{9,11,13,17} (4 alike) : DataTypeConversion  OutDataTypeStr=int8  SaturateOnIntegerOverflow=off  RndMeth=Floor
  Data Type Conversion12 : DataTypeConversion  OutDataTypeStr=int16  SaturateOnIntegerOverflow=off  RndMeth=Floor
  Data Type Conversion{2..3,5..8,14..16,18} (10 alike) : DataTypeConversion  OutDataTypeStr=single  SaturateOnIntegerOverflow=off  RndMeth=Floor
  Data Type Conversion4 : DataTypeConversion  OutDataTypeStr=uint8  SaturateOnIntegerOverflow=off  RndMeth=Floor
  VR_ADCU_IPM_Obj_20_0x663FromOutData : Outport  OutDataTypeStr=Bus:VR_ADCU_IPM_Obj_20_0x663
  wires:
  CAN FD Unpack/1 -> Data Type Conversion1/1
  CAN FD Unpack/2 -> Data Type Conversion2/1
  CAN FD Unpack/3 -> Data Type Conversion3/1
  CAN FD Unpack/4 -> Data Type Conversion4/1
  CAN FD Unpack/5 -> Data Type Conversion5/1
  CAN FD Unpack/6 -> Data Type Conversion6/1
  CAN FD Unpack/7 -> Data Type Conversion7/1
  CAN FD Unpack/8 -> Data Type Conversion8/1
  CAN FD Unpack/9 -> Data Type Conversion9/1
  CAN FD Unpack/10 -> Data Type Conversion10/1
  CAN FD Unpack/11 -> Data Type Conversion11/1
  CAN FD Unpack/12 -> Data Type Conversion12/1
  CAN FD Unpack/13 -> Data Type Conversion13/1
  CAN FD Unpack/14 -> Data Type Conversion14/1
  CAN FD Unpack/15 -> Data Type Conversion15/1
  CAN FD Unpack/16 -> Data Type Conversion16/1
  CAN FD Unpack/17 -> Data Type Conversion17/1
  CAN FD Unpack/18 -> Data Type Conversion18/1
  Data Type Conversion1/1 -> Bus Creator/1  "IPM_ObjBlockCounter_20"
  Data Type Conversion2/1 -> Bus Creator/2  "IPM_ObjDistX_20"
  Data Type Conversion3/1 -> Bus Creator/3  "IPM_ObjDistY_20"
  Data Type Conversion4/1 -> Bus Creator/4  "IPM_ObjID_20"
  Data Type Conversion5/1 -> Bus Creator/5  "IPM_ObjRelAccelX_20"
  Data Type Conversion6/1 -> Bus Creator/6  "IPM_ObjRelAccelY_20"
  Data Type Conversion7/1 -> Bus Creator/7  "IPM_ObjRelVelX_20"
  Data Type Conversion8/1 -> Bus Creator/8  "IPM_ObjRelVelY_20"
  Data Type Conversion9/1 -> Bus Creator/9  "IPM_ObjType_20"
  Data Type Conversion10/1 -> Bus Creator/10  "IPM_Obj_20_Checksum"
  Data Type Conversion11/1 -> Bus Creator/11  "IPM_Obj_20_MsgCounter"
  Data Type Conversion12/1 -> Bus Creator/12  "IPM_Object_Age_20"
  Data Type Conversion13/1 -> Bus Creator/13  "IPM_Object_Existence_Probability_20"
  Data Type Conversion14/1 -> Bus Creator/14  "IPM_Object_Heading_20"
  Data Type Conversion15/1 -> Bus Creator/15  "IPM_Object_Height_20"
  Data Type Conversion16/1 -> Bus Creator/16  "IPM_Object_Length_20"
  Data Type Conversion17/1 -> Bus Creator/17  "IPM_Object_Motion_Status_20"
  Data Type Conversion18/1 -> Bus Creator/18  "IPM_Object_Width_20"
  Bus Creator/1 -> VR_ADCU_IPM_Obj_20_0x663FromOutData/1  "VR_ADCU_IPM_Obj_20_0x663FromOutData"
  VR_ADCU_IPM_Obj_20_0x663FromInData/1 -> CAN FD Unpack/1  "VR_ADCU_IPM_Obj_20_0x663FromInData"

== system ALL_JP360_DBW_V6_5_1103/MsgFromCAN/VR_ADCU_MsgFromCAN/VR_ADCU_IPM_RightLine_0x590 ==
  VR_ADCU_IPM_RightLine_0x590FromInData : Inport  OutDataTypeStr=Bus:CAN_FD_MESSAGE_BUS
  Bus Creator : BusCreator  Inputs=6  OutDataTypeStr=Bus:VR_ADCU_IPM_RightLine_0x590  NonVirtualBus=on
  CAN FD Unpack : canfdmsglib/CAN FD Unpack  CANdbFile=HiFire_T360_P789_1R1V_Pri_Matrix_CAN_V2.3_20220810.dbc  MsgList=(none)  MsgName=IPM_RightLine_0x590  ProtocolMode=CAN FD  MsgIDType=Standard (11-bit identifier)  MsgIdentifier=1424  MsgLength=8  SignalInfo={'IPM_RightLine_dx_lookhead','27','9','BE','unsigned','Standard','0','0.25','0','0','127.75';'IPM_RightLine_dx_start','0','8','BE','unsigned','Standard','0','0.25','0','0','63.75';'IPM_RightLine_dy','20','12','BE','unsigned','Standard','0','0.0039062','-8','-8','7.9961';'IPM_RightLine_hor_curvature_alteration','58','10','BE','unsigned','Standard','0','0.0001','-0.015','-0.015','0.0873';'IPM_RightLine_hor_curve','33','10','BE','unsigned','Standard','0','0.0001','-0.015','-0.015','0.0873';'IPM_RightLine_yawangle','52','12','BE','unsigned','Standard','0','0.00048828','-1','-1','0.99951'}  IDPort=off  TimestampPort=off  ErrorPort=off  RemotePort=off  LengthPort=off  StatusPort=off  BRSPort=off  ESIPort=off  DLCPort=off  ApplyMinMax=off
      settings: SourceProductBaseCode=ME,XP,VN  DataFormat=CANdb specified signals
  Data Type Conversion{1..6} (6 alike) : DataTypeConversion  OutDataTypeStr=single  SaturateOnIntegerOverflow=off  RndMeth=Floor
  VR_ADCU_IPM_RightLine_0x590FromOutData : Outport  OutDataTypeStr=Bus:VR_ADCU_IPM_RightLine_0x590
  wires:
  CAN FD Unpack/1 -> Data Type Conversion1/1
  CAN FD Unpack/2 -> Data Type Conversion2/1
  CAN FD Unpack/3 -> Data Type Conversion3/1
  CAN FD Unpack/4 -> Data Type Conversion4/1
  CAN FD Unpack/5 -> Data Type Conversion5/1
  CAN FD Unpack/6 -> Data Type Conversion6/1
  Data Type Conversion1/1 -> Bus Creator/1  "IPM_RightLine_dx_lookhead"
  Data Type Conversion2/1 -> Bus Creator/2  "IPM_RightLine_dx_start"
  Data Type Conversion3/1 -> Bus Creator/3  "IPM_RightLine_dy"
  Data Type Conversion4/1 -> Bus Creator/4  "IPM_RightLine_hor_curvature_alteration"
  Data Type Conversion5/1 -> Bus Creator/5  "IPM_RightLine_hor_curve"
  Data Type Conversion6/1 -> Bus Creator/6  "IPM_RightLine_yawangle"
  Bus Creator/1 -> VR_ADCU_IPM_RightLine_0x590FromOutData/1  "VR_ADCU_IPM_RightLine_0x590FromOutData"
  VR_ADCU_IPM_RightLine_0x590FromInData/1 -> CAN FD Unpack/1  "VR_ADCU_IPM_RightLine_0x590FromInData"

== system ALL_JP360_DBW_V6_5_1103/MsgFromCAN/VR_ADCU_MsgFromCAN/VR_ADCU_IPM_RightLine_0x591 ==
  VR_ADCU_IPM_RightLine_0x591FromInData : Inport  OutDataTypeStr=Bus:CAN_FD_MESSAGE_BUS
  Bus Creator : BusCreator  Inputs=9  OutDataTypeStr=Bus:VR_ADCU_IPM_RightLine_0x591  NonVirtualBus=on
  CAN FD Unpack : canfdmsglib/CAN FD Unpack  CANdbFile=HiFire_T360_P789_1R1V_Pri_Matrix_CAN_V2.3_20220810.dbc  MsgList=(none)  MsgName=IPM_RightLine_0x591  ProtocolMode=CAN FD  MsgIDType=Standard (11-bit identifier)  MsgIdentifier=1425  MsgLength=8  SignalInfo={'IPM_LineAssit_RightRightVisualization','0','2','BE','unsigned','Standard','0','1','0','0','3';'IPM_RighRightLine_Color','13','3','BE','unsigned','Standard','0','1','0','0','7';'IPM_RightLine_Color','5','3','BE','unsigned','Standard','0','1','0','0','7';'IPM_RightLine_Type','2','3','BE','unsigned','Standard','0','1','0','0','7';'IPM_RightRighLine_Type','10','3','BE','unsigned','Standard','0','1','0','0','7';'IPM_RightRightLine_curvature_alteration','56','12','BE','unsigned','Standard','0','0.0001','-0.015','-0.015','0.0873';'IPM_RightRightLine_dy','28','12','BE','unsigned','Standard','0','0.0039062','-8','-8','7.9961';'IPM_RightRightLine_hor_curve','33','10','BE','unsigned','Standard','0','0.0001','-0.015','-0.015','0.0873';'IPM_RightRightLine_yawangle','52','12','BE','unsigned','Standard','0','0.00048828','-1','-1','0.99951'}  IDPort=off  TimestampPort=off  ErrorPort=off  RemotePort=off  LengthPort=off  StatusPort=off  BRSPort=off  ESIPort=off  DLCPort=off  ApplyMinMax=off
      settings: SourceProductBaseCode=ME,XP,VN  DataFormat=CANdb specified signals
  Data Type Conversion{1..5} (5 alike) : DataTypeConversion  OutDataTypeStr=int8  SaturateOnIntegerOverflow=off  RndMeth=Floor
  Data Type Conversion{6..9} (4 alike) : DataTypeConversion  OutDataTypeStr=single  SaturateOnIntegerOverflow=off  RndMeth=Floor
  VR_ADCU_IPM_RightLine_0x591FromOutData : Outport  OutDataTypeStr=Bus:VR_ADCU_IPM_RightLine_0x591
  wires:
  CAN FD Unpack/1 -> Data Type Conversion1/1
  CAN FD Unpack/2 -> Data Type Conversion2/1
  CAN FD Unpack/3 -> Data Type Conversion3/1
  CAN FD Unpack/4 -> Data Type Conversion4/1
  CAN FD Unpack/5 -> Data Type Conversion5/1
  CAN FD Unpack/6 -> Data Type Conversion6/1
  CAN FD Unpack/7 -> Data Type Conversion7/1
  CAN FD Unpack/8 -> Data Type Conversion8/1
  CAN FD Unpack/9 -> Data Type Conversion9/1
  Data Type Conversion1/1 -> Bus Creator/1  "IPM_LineAssit_RightRightVisualization"
  Data Type Conversion2/1 -> Bus Creator/2  "IPM_RighRightLine_Color"
  Data Type Conversion3/1 -> Bus Creator/3  "IPM_RightLine_Color"
  Data Type Conversion4/1 -> Bus Creator/4  "IPM_RightLine_Type"
  Data Type Conversion5/1 -> Bus Creator/5  "IPM_RightRighLine_Type"
  Data Type Conversion6/1 -> Bus Creator/6  "IPM_RightRightLine_curvature_alteration"
  Data Type Conversion7/1 -> Bus Creator/7  "IPM_RightRightLine_dy"
  Data Type Conversion8/1 -> Bus Creator/8  "IPM_RightRightLine_hor_curve"
  Data Type Conversion9/1 -> Bus Creator/9  "IPM_RightRightLine_yawangle"
  Bus Creator/1 -> VR_ADCU_IPM_RightLine_0x591FromOutData/1  "VR_ADCU_IPM_RightLine_0x591FromOutData"
  VR_ADCU_IPM_RightLine_0x591FromInData/1 -> CAN FD Unpack/1  "VR_ADCU_IPM_RightLine_0x591FromInData"
